simulink library "mylib"  (R2020a)
settings: Solver=VariableStepAuto  StartTime=0.0  StopTime=10.0  RelTol=1e-3
undefined symbols (not defined in the file): d_du_max_pu, dir_to_bus1, dir_to_bus_0L, dir_to_bus_2, dir_to_line1, dir_to_line_0L, dir_to_line_2, du_max_pu, du_ph_max_pu, Fi_0, Fi_T_H, Fi_T_L, Fi_T_M, I0_calc_0L, I0_comp_H, I0_comp_L, I0_comp_M, I0_max_0L, I2_max_2, I_diff1, I_diff2, I_diff3, I_diff4, I_diff5, I_diff_to, I_hight_CT1_G, I_hight_CT2_G, I_low_CT1, I_low_CT2, I_max1, I_max2, I_max3, I_max4, I_max5, I_min_sec_CT1, I_min_sec_CT2, I_unb, Iph_max_0L, Iph_max_2, jmp_in_zone, jmp_in_zone_0L, jmp_in_zone_2, K_dop, max_min1, only_K1_0L, only_K1_2, only_K2_0L, only_K2_2, only_K3_0L, only_K3_2, P_ctl_0, PQ_Fi_ctl_0, Q_ctl_0, S_set_0, set, set1, T_fast, T_I_ctl, T_off, T_on ... (+15)
libraries: $bdroot x184, powerlib_meascontrol x97
(part 6 of 14)

== system mylib/262_tnznp_line_st_v1/230_st18_ph/k_type ==
  In_a : Inport
  In_b : Inport  Port=2
  In_ c : Inport  Port=3
  only_K1 : Inport  Port=4
  only_K2 : Inport  Port=5
  only_K3 : Inport  Port=6
  1 : Switch  Criteria=u2 > Threshold
  Logical Operator{1,12,18..27} (12 alike) : Logic  Operator=NOT  AllPortsSameDT=off  OutDataTypeStr=boolean
  Logical Operator10 : Logic  AllPortsSameDT=off  OutDataTypeStr=boolean
  Logical Operator{2..4,7..8,11,14,17} (8 alike) : Logic  Inputs=3  AllPortsSameDT=off  OutDataTypeStr=boolean
  Logical Operator{5..6,13,16} (4 alike) : Logic  Operator=OR  Inputs=3  AllPortsSameDT=off  OutDataTypeStr=boolean
  Logical Operator15 : Logic  AllPortsSameDT=off  OutDataTypeStr=boolean
  Logical Operator9 : Logic  AllPortsSameDT=off  OutDataTypeStr=boolean
  out : Outport
  wires:
  In_ c/1 -> Logical Operator14/3, Logical Operator16/3, Logical Operator21/1, Logical Operator7/3, Logical Operator4/3, Logical Operator3/3, Logical Operator25/1, Logical Operator1/1
  Logical Operator16/1 -> 1/1
  Logical Operator13/1 -> 1/3
  1/1 -> out/1
  Logical Operator17/1 -> 1/2
  only_K3/1 -> Logical Operator20/1, Logical Operator15/1
  only_K2/1 -> Logical Operator10/1, Logical Operator18/1
  only_K1/1 -> Logical Operator9/1, Logical Operator19/1
  In_b/1 -> Logical Operator14/2, Logical Operator16/2, Logical Operator8/2, Logical Operator22/1, Logical Operator4/2, Logical Operator27/1, Logical Operator2/2, Logical Operator12/1
  Logical Operator27/1 -> Logical Operator3/2
  Logical Operator26/1 -> Logical Operator3/1
  Logical Operator25/1 -> Logical Operator2/3
  In_a/1 -> Logical Operator11/1, Logical Operator24/1, Logical Operator14/1, Logical Operator16/1, Logical Operator8/1, Logical Operator7/1, Logical Operator23/1, Logical Operator26/1
  Logical Operator24/1 -> Logical Operator2/1
  Logical Operator23/1 -> Logical Operator4/1
  Logical Operator22/1 -> Logical Operator7/2
  Logical Operator21/1 -> Logical Operator8/3
  Logical Operator20/1 -> Logical Operator17/3
  Logical Operator18/1 -> Logical Operator17/2
  Logical Operator19/1 -> Logical Operator17/1
  Logical Operator14/1 -> Logical Operator15/2
  Logical Operator15/1 -> Logical Operator13/3
  Logical Operator10/1 -> Logical Operator13/2
  Logical Operator9/1 -> Logical Operator13/1
  Logical Operator6/1 -> Logical Operator10/2
  Logical Operator5/1 -> Logical Operator9/2
  Logical Operator8/1 -> Logical Operator6/3
  Logical Operator7/1 -> Logical Operator6/2
  Logical Operator4/1 -> Logical Operator6/1
  Logical Operator3/1 -> Logical Operator5/3
  Logical Operator11/1 -> Logical Operator5/1
  Logical Operator2/1 -> Logical Operator5/2
  Logical Operator1/1 -> Logical Operator11/3
  Logical Operator12/1 -> Logical Operator11/2

== system mylib/264_DZ_trans_st_v1/Poly12_det19_ph/Za ==
  re : Inport
  im : Inport  Port=2
  Re1 : Inport  Port=3
  Im1 : Inport  Port=4
  Re2 : Inport  Port=5
  Im2 : Inport  Port=6
  Re3 : Inport  Port=7
  Im3 : Inport  Port=8
  Re4 : Inport  Port=9
  Im4 : Inport  Port=10
  Re5 : Inport  Port=11
  Im5 : Inport  Port=12
  Re6 : Inport  Port=13
  Im6 : Inport  Port=14
  Re7 : Inport  Port=15
  Im7 : Inport  Port=16
  Re8 : Inport  Port=17
  Im8 : Inport  Port=18
  Re9 : Inport  Port=19
  Im9 : Inport  Port=20
  Re10 : Inport  Port=21
  Im10 : Inport  Port=22
  Re11 : Inport  Port=23
  Im11 : Inport  Port=24
  Re12 : Inport  Port=25
  Im12 : Inport  Port=26
  Constant : Constant  Value=0
  Logical Operator : Logic  Operator=NOT  AllPortsSameDT=off  OutDataTypeStr=boolean
  Logical Operator1 : Logic  Operator=NOT  AllPortsSameDT=off  OutDataTypeStr=boolean
  stp_1 : Subsystem
  stp_10 : Subsystem
  stp_11 : Subsystem
  stp_12 : Subsystem
  stp_2 : Subsystem
  stp_3 : Subsystem
  stp_4 : Subsystem
  stp_5 : Subsystem
  stp_6 : Subsystem
  stp_7 : Subsystem
  stp_8 : Subsystem
  stp_9 : Subsystem
  Y : Outport
  not_Y : Outport  Port=2
  wires:
  Logical Operator/1 -> stp_1/9(start_pt)
  Constant/1 -> stp_1/1(Y_in), stp_1/2(alg_in), Logical Operator/1, stp_2/9(start_pt), stp_12/9(start_pt), stp_11/9(start_pt), stp_10/9(start_pt), stp_9/9(start_pt), stp_8/9(start_pt), stp_7/9(start_pt), stp_6/9(start_pt), stp_5/9(start_pt), stp_4/9(start_pt), stp_3/9(start_pt)
  stp_1/4(cur_Im) -> stp_2/4(Im_cur)
  stp_1/3(cur_Re) -> stp_2/3(Re_cur)
  stp_1/2(alg_out) -> stp_2/2(alg_in)
  stp_1/1(Y_out) -> stp_2/1(Y_in)
  im/1 -> stp_12/8(im), stp_11/8(im), stp_10/8(im), stp_9/8(im), stp_8/8(im), stp_7/8(im), stp_6/8(im), stp_5/8(im), stp_4/8(im), stp_3/8(im), stp_2/8(im), stp_1/8(im)
  re/1 -> stp_12/7(re), stp_11/7(re), stp_10/7(re), stp_9/7(re), stp_8/7(re), stp_7/7(re), stp_6/7(re), stp_5/7(re), stp_4/7(re), stp_3/7(re), stp_2/7(re), stp_1/7(re)
  Re1/1 -> stp_1/3(Re_cur), stp_1/10(Re_start), stp_12/5(Re_next), stp_12/10(Re_start), stp_11/10(Re_start), stp_10/10(Re_start), stp_9/10(Re_start), stp_8/10(Re_start), stp_7/10(Re_start), stp_6/10(Re_start), stp_5/10(Re_start), stp_4/10(Re_start), stp_3/10(Re_start), stp_2/10(Re_start)
  Im1/1 -> stp_1/4(Im_cur), stp_1/11(Im_start), stp_12/6(Im_next), stp_12/11(Im_start), stp_11/11(Im_start), stp_10/11(Im_start), stp_9/11(Im_start), stp_8/11(Im_start), stp_7/11(Im_start), stp_6/11(Im_start), stp_5/11(Im_start), stp_4/11(Im_start), stp_3/11(Im_start), stp_2/11(Im_start)
  Re2/1 -> stp_1/5(Re_next)
  Im2/1 -> stp_1/6(Im_next)
  Re3/1 -> stp_2/5(Re_next)
  Im3/1 -> stp_2/6(Im_next)
  Re4/1 -> stp_3/5(Re_next)
  Im4/1 -> stp_3/6(Im_next)
  stp_2/1(Y_out) -> stp_3/1(Y_in)
  stp_2/2(alg_out) -> stp_3/2(alg_in)
  stp_2/3(cur_Re) -> stp_3/3(Re_cur)
  stp_2/4(cur_Im) -> stp_3/4(Im_cur)
  stp_10/1(Y_out) -> stp_11/1(Y_in)
  stp_10/2(alg_out) -> stp_11/2(alg_in)
  stp_10/3(cur_Re) -> stp_11/3(Re_cur)
  stp_10/4(cur_Im) -> stp_11/4(Im_cur)
  stp_11/1(Y_out) -> stp_12/1(Y_in)
  stp_11/2(alg_out) -> stp_12/2(alg_in)
  stp_11/3(cur_Re) -> stp_12/3(Re_cur)
  stp_11/4(cur_Im) -> stp_12/4(Im_cur)
  stp_9/4(cur_Im) -> stp_10/4(Im_cur)
  stp_9/3(cur_Re) -> stp_10/3(Re_cur)
  stp_9/2(alg_out) -> stp_10/2(alg_in)
  stp_9/1(Y_out) -> stp_10/1(Y_in)
  stp_8/4(cur_Im) -> stp_9/4(Im_cur)
  stp_8/3(cur_Re) -> stp_9/3(Re_cur)
  stp_8/2(alg_out) -> stp_9/2(alg_in)
  stp_8/1(Y_out) -> stp_9/1(Y_in)
  stp_7/4(cur_Im) -> stp_8/4(Im_cur)
  stp_7/3(cur_Re) -> stp_8/3(Re_cur)
  stp_7/2(alg_out) -> stp_8/2(alg_in)
  stp_7/1(Y_out) -> stp_8/1(Y_in)
  stp_6/4(cur_Im) -> stp_7/4(Im_cur)
  stp_6/3(cur_Re) -> stp_7/3(Re_cur)
  stp_6/2(alg_out) -> stp_7/2(alg_in)
  stp_6/1(Y_out) -> stp_7/1(Y_in)
  stp_5/4(cur_Im) -> stp_6/4(Im_cur)
  stp_5/3(cur_Re) -> stp_6/3(Re_cur)
  stp_5/2(alg_out) -> stp_6/2(alg_in)
  stp_5/1(Y_out) -> stp_6/1(Y_in)
  stp_4/4(cur_Im) -> stp_5/4(Im_cur)
  stp_4/3(cur_Re) -> stp_5/3(Re_cur)
  stp_4/2(alg_out) -> stp_5/2(alg_in)
  stp_4/1(Y_out) -> stp_5/1(Y_in)
  stp_3/4(cur_Im) -> stp_4/4(Im_cur)
  stp_3/3(cur_Re) -> stp_4/3(Re_cur)
  stp_3/2(alg_out) -> stp_4/2(alg_in)
  stp_3/1(Y_out) -> stp_4/1(Y_in)
  Re5/1 -> stp_4/5(Re_next)
  Im5/1 -> stp_4/6(Im_next)
  Re6/1 -> stp_5/5(Re_next)
  Im6/1 -> stp_5/6(Im_next)
  Re7/1 -> stp_6/5(Re_next)
  Im7/1 -> stp_6/6(Im_next)
  Re8/1 -> stp_7/5(Re_next)
  Im8/1 -> stp_7/6(Im_next)
  Re9/1 -> stp_8/5(Re_next)
  Im9/1 -> stp_8/6(Im_next)
  Re10/1 -> stp_9/5(Re_next)
  Im10/1 -> stp_9/6(Im_next)
  Re11/1 -> stp_10/5(Re_next)
  Im11/1 -> stp_10/6(Im_next)
  Re12/1 -> stp_11/5(Re_next)
  Im12/1 -> stp_11/6(Im_next)
  stp_12/1(Y_out) -> Logical Operator1/1, Y/1
  Logical Operator1/1 -> not_Y/1

== system mylib/264_DZ_trans_st_v1/Poly12_det19_ph/Zb ==
  re : Inport
  im : Inport  Port=2
  Re1 : Inport  Port=3
  Im1 : Inport  Port=4
  Re2 : Inport  Port=5
  Im2 : Inport  Port=6
  Re3 : Inport  Port=7
  Im3 : Inport  Port=8
  Re4 : Inport  Port=9
  Im4 : Inport  Port=10
  Re5 : Inport  Port=11
  Im5 : Inport  Port=12
  Re6 : Inport  Port=13
  Im6 : Inport  Port=14
  Re7 : Inport  Port=15
  Im7 : Inport  Port=16
  Re8 : Inport  Port=17
  Im8 : Inport  Port=18
  Re9 : Inport  Port=19
  Im9 : Inport  Port=20
  Re10 : Inport  Port=21
  Im10 : Inport  Port=22
  Re11 : Inport  Port=23
  Im11 : Inport  Port=24
  Re12 : Inport  Port=25
  Im12 : Inport  Port=26
  Constant : Constant  Value=0
  Logical Operator : Logic  Operator=NOT  AllPortsSameDT=off  OutDataTypeStr=boolean
  Logical Operator1 : Logic  Operator=NOT  AllPortsSameDT=off  OutDataTypeStr=boolean
  stp_1 : Subsystem
  stp_10 : Subsystem
  stp_11 : Subsystem
  stp_12 : Subsystem
  stp_2 : Subsystem
  stp_3 : Subsystem
  stp_4 : Subsystem
  stp_5 : Subsystem
  stp_6 : Subsystem
  stp_7 : Subsystem
  stp_8 : Subsystem
  stp_9 : Subsystem
  Y : Outport
  not_Y : Outport  Port=2
  wires:
  Logical Operator/1 -> stp_1/9(start_pt)
  Constant/1 -> stp_1/1(Y_in), stp_1/2(alg_in), Logical Operator/1, stp_2/9(start_pt), stp_12/9(start_pt), stp_11/9(start_pt), stp_10/9(start_pt), stp_9/9(start_pt), stp_8/9(start_pt), stp_7/9(start_pt), stp_6/9(start_pt), stp_5/9(start_pt), stp_4/9(start_pt), stp_3/9(start_pt)
  stp_1/4(cur_Im) -> stp_2/4(Im_cur)
  stp_1/3(cur_Re) -> stp_2/3(Re_cur)
  stp_1/2(alg_out) -> stp_2/2(alg_in)
  stp_1/1(Y_out) -> stp_2/1(Y_in)
  im/1 -> stp_12/8(im), stp_11/8(im), stp_10/8(im), stp_9/8(im), stp_8/8(im), stp_7/8(im), stp_6/8(im), stp_5/8(im), stp_4/8(im), stp_3/8(im), stp_2/8(im), stp_1/8(im)
  re/1 -> stp_12/7(re), stp_11/7(re), stp_10/7(re), stp_9/7(re), stp_8/7(re), stp_7/7(re), stp_6/7(re), stp_5/7(re), stp_4/7(re), stp_3/7(re), stp_2/7(re), stp_1/7(re)
  Re1/1 -> stp_1/3(Re_cur), stp_1/10(Re_start), stp_12/5(Re_next), stp_12/10(Re_start), stp_11/10(Re_start), stp_10/10(Re_start), stp_9/10(Re_start), stp_8/10(Re_start), stp_7/10(Re_start), stp_6/10(Re_start), stp_5/10(Re_start), stp_4/10(Re_start), stp_3/10(Re_start), stp_2/10(Re_start)
  Im1/1 -> stp_1/4(Im_cur), stp_1/11(Im_start), stp_12/6(Im_next), stp_12/11(Im_start), stp_11/11(Im_start), stp_10/11(Im_start), stp_9/11(Im_start), stp_8/11(Im_start), stp_7/11(Im_start), stp_6/11(Im_start), stp_5/11(Im_start), stp_4/11(Im_start), stp_3/11(Im_start), stp_2/11(Im_start)
  Re2/1 -> stp_1/5(Re_next)
  Im2/1 -> stp_1/6(Im_next)
  Re3/1 -> stp_2/5(Re_next)
  Im3/1 -> stp_2/6(Im_next)
  Re4/1 -> stp_3/5(Re_next)
  Im4/1 -> stp_3/6(Im_next)
  stp_2/1(Y_out) -> stp_3/1(Y_in)
  stp_2/2(alg_out) -> stp_3/2(alg_in)
  stp_2/3(cur_Re) -> stp_3/3(Re_cur)
  stp_2/4(cur_Im) -> stp_3/4(Im_cur)
  stp_10/1(Y_out) -> stp_11/1(Y_in)
  stp_10/2(alg_out) -> stp_11/2(alg_in)
  stp_10/3(cur_Re) -> stp_11/3(Re_cur)
  stp_10/4(cur_Im) -> stp_11/4(Im_cur)
  stp_11/1(Y_out) -> stp_12/1(Y_in)
  stp_11/2(alg_out) -> stp_12/2(alg_in)
  stp_11/3(cur_Re) -> stp_12/3(Re_cur)
  stp_11/4(cur_Im) -> stp_12/4(Im_cur)
  stp_9/4(cur_Im) -> stp_10/4(Im_cur)
  stp_9/3(cur_Re) -> stp_10/3(Re_cur)
  stp_9/2(alg_out) -> stp_10/2(alg_in)
  stp_9/1(Y_out) -> stp_10/1(Y_in)
  stp_8/4(cur_Im) -> stp_9/4(Im_cur)
  stp_8/3(cur_Re) -> stp_9/3(Re_cur)
  stp_8/2(alg_out) -> stp_9/2(alg_in)
  stp_8/1(Y_out) -> stp_9/1(Y_in)
  stp_7/4(cur_Im) -> stp_8/4(Im_cur)
  stp_7/3(cur_Re) -> stp_8/3(Re_cur)
  stp_7/2(alg_out) -> stp_8/2(alg_in)
  stp_7/1(Y_out) -> stp_8/1(Y_in)
  stp_6/4(cur_Im) -> stp_7/4(Im_cur)
  stp_6/3(cur_Re) -> stp_7/3(Re_cur)
  stp_6/2(alg_out) -> stp_7/2(alg_in)
  stp_6/1(Y_out) -> stp_7/1(Y_in)
  stp_5/4(cur_Im) -> stp_6/4(Im_cur)
  stp_5/3(cur_Re) -> stp_6/3(Re_cur)
  stp_5/2(alg_out) -> stp_6/2(alg_in)
  stp_5/1(Y_out) -> stp_6/1(Y_in)
  stp_4/4(cur_Im) -> stp_5/4(Im_cur)
  stp_4/3(cur_Re) -> stp_5/3(Re_cur)
  stp_4/2(alg_out) -> stp_5/2(alg_in)
  stp_4/1(Y_out) -> stp_5/1(Y_in)
  stp_3/4(cur_Im) -> stp_4/4(Im_cur)
  stp_3/3(cur_Re) -> stp_4/3(Re_cur)
  stp_3/2(alg_out) -> stp_4/2(alg_in)
  stp_3/1(Y_out) -> stp_4/1(Y_in)
  Re5/1 -> stp_4/5(Re_next)
  Im5/1 -> stp_4/6(Im_next)
  Re6/1 -> stp_5/5(Re_next)
  Im6/1 -> stp_5/6(Im_next)
  Re7/1 -> stp_6/5(Re_next)
  Im7/1 -> stp_6/6(Im_next)
  Re8/1 -> stp_7/5(Re_next)
  Im8/1 -> stp_7/6(Im_next)
  Re9/1 -> stp_8/5(Re_next)
  Im9/1 -> stp_8/6(Im_next)
  Re10/1 -> stp_9/5(Re_next)
  Im10/1 -> stp_9/6(Im_next)
  Re11/1 -> stp_10/5(Re_next)
  Im11/1 -> stp_10/6(Im_next)
  Re12/1 -> stp_11/5(Re_next)
  Im12/1 -> stp_11/6(Im_next)
  stp_12/1(Y_out) -> Logical Operator1/1, Y/1
  Logical Operator1/1 -> not_Y/1

== system mylib/264_DZ_trans_st_v1/Poly12_det19_ph/Zc ==
  re : Inport
  im : Inport  Port=2
  Re1 : Inport  Port=3
  Im1 : Inport  Port=4
  Re2 : Inport  Port=5
  Im2 : Inport  Port=6
  Re3 : Inport  Port=7
  Im3 : Inport  Port=8
  Re4 : Inport  Port=9
  Im4 : Inport  Port=10
  Re5 : Inport  Port=11
  Im5 : Inport  Port=12
  Re6 : Inport  Port=13
  Im6 : Inport  Port=14
  Re7 : Inport  Port=15
  Im7 : Inport  Port=16
  Re8 : Inport  Port=17
  Im8 : Inport  Port=18
  Re9 : Inport  Port=19
  Im9 : Inport  Port=20
  Re10 : Inport  Port=21
  Im10 : Inport  Port=22
  Re11 : Inport  Port=23
  Im11 : Inport  Port=24
  Re12 : Inport  Port=25
  Im12 : Inport  Port=26
  Constant : Constant  Value=0
  Logical Operator : Logic  Operator=NOT  AllPortsSameDT=off  OutDataTypeStr=boolean
  Logical Operator1 : Logic  Operator=NOT  AllPortsSameDT=off  OutDataTypeStr=boolean
  stp_1 : Subsystem
  stp_10 : Subsystem
  stp_11 : Subsystem
  stp_12 : Subsystem
  stp_2 : Subsystem
  stp_3 : Subsystem
  stp_4 : Subsystem
  stp_5 : Subsystem
  stp_6 : Subsystem
  stp_7 : Subsystem
  stp_8 : Subsystem
  stp_9 : Subsystem
  Y : Outport
  not_Y : Outport  Port=2
  wires:
  Logical Operator/1 -> stp_1/9(start_pt)
  Constant/1 -> stp_1/1(Y_in), stp_1/2(alg_in), Logical Operator/1, stp_2/9(start_pt), stp_12/9(start_pt), stp_11/9(start_pt), stp_10/9(start_pt), stp_9/9(start_pt), stp_8/9(start_pt), stp_7/9(start_pt), stp_6/9(start_pt), stp_5/9(start_pt), stp_4/9(start_pt), stp_3/9(start_pt)
  stp_1/4(cur_Im) -> stp_2/4(Im_cur)
  stp_1/3(cur_Re) -> stp_2/3(Re_cur)
  stp_1/2(alg_out) -> stp_2/2(alg_in)
  stp_1/1(Y_out) -> stp_2/1(Y_in)
  im/1 -> stp_12/8(im), stp_11/8(im), stp_10/8(im), stp_9/8(im), stp_8/8(im), stp_7/8(im), stp_6/8(im), stp_5/8(im), stp_4/8(im), stp_3/8(im), stp_2/8(im), stp_1/8(im)
  re/1 -> stp_12/7(re), stp_11/7(re), stp_10/7(re), stp_9/7(re), stp_8/7(re), stp_7/7(re), stp_6/7(re), stp_5/7(re), stp_4/7(re), stp_3/7(re), stp_2/7(re), stp_1/7(re)
  Re1/1 -> stp_1/3(Re_cur), stp_1/10(Re_start), stp_12/5(Re_next), stp_12/10(Re_start), stp_11/10(Re_start), stp_10/10(Re_start), stp_9/10(Re_start), stp_8/10(Re_start), stp_7/10(Re_start), stp_6/10(Re_start), stp_5/10(Re_start), stp_4/10(Re_start), stp_3/10(Re_start), stp_2/10(Re_start)
  Im1/1 -> stp_1/4(Im_cur), stp_1/11(Im_start), stp_12/6(Im_next), stp_12/11(Im_start), stp_11/11(Im_start), stp_10/11(Im_start), stp_9/11(Im_start), stp_8/11(Im_start), stp_7/11(Im_start), stp_6/11(Im_start), stp_5/11(Im_start), stp_4/11(Im_start), stp_3/11(Im_start), stp_2/11(Im_start)
  Re2/1 -> stp_1/5(Re_next)
  Im2/1 -> stp_1/6(Im_next)
  Re3/1 -> stp_2/5(Re_next)
  Im3/1 -> stp_2/6(Im_next)
  Re4/1 -> stp_3/5(Re_next)
  Im4/1 -> stp_3/6(Im_next)
  stp_2/1(Y_out) -> stp_3/1(Y_in)
  stp_2/2(alg_out) -> stp_3/2(alg_in)
  stp_2/3(cur_Re) -> stp_3/3(Re_cur)
  stp_2/4(cur_Im) -> stp_3/4(Im_cur)
  stp_10/1(Y_out) -> stp_11/1(Y_in)
  stp_10/2(alg_out) -> stp_11/2(alg_in)
  stp_10/3(cur_Re) -> stp_11/3(Re_cur)
  stp_10/4(cur_Im) -> stp_11/4(Im_cur)
  stp_11/1(Y_out) -> stp_12/1(Y_in)
  stp_11/2(alg_out) -> stp_12/2(alg_in)
  stp_11/3(cur_Re) -> stp_12/3(Re_cur)
  stp_11/4(cur_Im) -> stp_12/4(Im_cur)
  stp_9/4(cur_Im) -> stp_10/4(Im_cur)
  stp_9/3(cur_Re) -> stp_10/3(Re_cur)
  stp_9/2(alg_out) -> stp_10/2(alg_in)
  stp_9/1(Y_out) -> stp_10/1(Y_in)
  stp_8/4(cur_Im) -> stp_9/4(Im_cur)
  stp_8/3(cur_Re) -> stp_9/3(Re_cur)
  stp_8/2(alg_out) -> stp_9/2(alg_in)
  stp_8/1(Y_out) -> stp_9/1(Y_in)
  stp_7/4(cur_Im) -> stp_8/4(Im_cur)
  stp_7/3(cur_Re) -> stp_8/3(Re_cur)
  stp_7/2(alg_out) -> stp_8/2(alg_in)
  stp_7/1(Y_out) -> stp_8/1(Y_in)
  stp_6/4(cur_Im) -> stp_7/4(Im_cur)
  stp_6/3(cur_Re) -> stp_7/3(Re_cur)
  stp_6/2(alg_out) -> stp_7/2(alg_in)
  stp_6/1(Y_out) -> stp_7/1(Y_in)
  stp_5/4(cur_Im) -> stp_6/4(Im_cur)
  stp_5/3(cur_Re) -> stp_6/3(Re_cur)
  stp_5/2(alg_out) -> stp_6/2(alg_in)
  stp_5/1(Y_out) -> stp_6/1(Y_in)
  stp_4/4(cur_Im) -> stp_5/4(Im_cur)
  stp_4/3(cur_Re) -> stp_5/3(Re_cur)
  stp_4/2(alg_out) -> stp_5/2(alg_in)
  stp_4/1(Y_out) -> stp_5/1(Y_in)
  stp_3/4(cur_Im) -> stp_4/4(Im_cur)
  stp_3/3(cur_Re) -> stp_4/3(Re_cur)
  stp_3/2(alg_out) -> stp_4/2(alg_in)
  stp_3/1(Y_out) -> stp_4/1(Y_in)
  Re5/1 -> stp_4/5(Re_next)
  Im5/1 -> stp_4/6(Im_next)
  Re6/1 -> stp_5/5(Re_next)
  Im6/1 -> stp_5/6(Im_next)
  Re7/1 -> stp_6/5(Re_next)
  Im7/1 -> stp_6/6(Im_next)
  Re8/1 -> stp_7/5(Re_next)
  Im8/1 -> stp_7/6(Im_next)
  Re9/1 -> stp_8/5(Re_next)
  Im9/1 -> stp_8/6(Im_next)
  Re10/1 -> stp_9/5(Re_next)
  Im10/1 -> stp_9/6(Im_next)
  Re11/1 -> stp_10/5(Re_next)
  Im11/1 -> stp_10/6(Im_next)
  Re12/1 -> stp_11/5(Re_next)
  Im12/1 -> stp_11/6(Im_next)
  stp_12/1(Y_out) -> Logical Operator1/1, Y/1
  Logical Operator1/1 -> not_Y/1

== system mylib/264_DZ_trans_st_v1/St1/Subsystem ==
  T_fast_time : Inport
  T_fast_zero : Inport  Port=2
  "In1 " : Inport  Port=3
  "In2 " : Inport  Port=4
  "In3 " : Inport  Port=5
  {1..5,7} (6 alike) : Switch  Criteria=u2 > Threshold
  T1 : powerlib_meascontrol/Logic/On Delay  DelayType=On delay  delay=T_st  ic=0  Ts=0
  T2 : powerlib_meascontrol/Logic/On Delay  DelayType=On delay  delay=T_st  ic=0  Ts=0
  T3 : powerlib_meascontrol/Logic/On Delay  DelayType=On delay  delay=T_st  ic=0  Ts=0
  T4 : powerlib_meascontrol/Logic/On Delay  DelayType=On delay  delay=T_fast  ic=0  Ts=0
  T5 : powerlib_meascontrol/Logic/On Delay  DelayType=On delay  delay=T_fast  ic=0  Ts=0
  T6 : powerlib_meascontrol/Logic/On Delay  DelayType=On delay  delay=T_fast  ic=0  Ts=0
  T7 : powerlib_meascontrol/Logic/On Delay  DelayType=Off delay  delay=T_fast  ic=0  Ts=0
  Out1 : Outport
  Out2 : Outport  Port=2
  Out3 : Outport  Port=3
  wires:
  "In3 "/1 -> T4/1, T2/1, 4/1
  "In2 "/1 -> 3/1, T5/1, T1/1
  "In1 "/1 -> 5/1, T3/1, T6/1
  T7/1 -> 2/2, 1/2, 7/2
  T_fast_time/1 -> T7/1
  T4/1 -> 2/1
  T5/1 -> 1/1
  T6/1 -> 7/1
  T3/1 -> 7/3
  T1/1 -> 1/3
  T2/1 -> 2/3
  T_fast_zero/1 -> 5/2, 3/2, 4/2
  7/1 -> 5/3
  1/1 -> 3/3
  2/1 -> 4/3
  5/1 -> Out1/1
  3/1 -> Out2/1
  4/1 -> Out3/1

== system mylib/264_DZ_trans_st_v1/St1/in_1 ==
  jmp_in_zone : Inport
  in : Inport  Port=2
  jmp : Inport  Port=3
  1 : Switch  Criteria=u2 > Threshold
  10 : Logic  AllPortsSameDT=off  OutDataTypeStr=boolean
  11 : Logic  Operator=NOT  AllPortsSameDT=off  OutDataTypeStr=boolean
  12 : Memory
  3 : Logic  AllPortsSameDT=off  OutDataTypeStr=boolean
  RS : $bdroot/RS  SystemSampleTime=-1  Latency=0  AutoFrameSizeCalculation=off
  R_TRIG : $bdroot/R_TRIG  SystemSampleTime=-1  Latency=0  AutoFrameSizeCalculation=off
  T1 : powerlib_meascontrol/Logic/On Delay  DelayType=Off delay  delay=T_reset  ic=0  Ts=0
  T2 : powerlib_meascontrol/Logic/On Delay  DelayType=On delay  delay=T_reset  ic=0  Ts=0
  Y : Outport
  wires:
  RS/1 -> 12/1, Y/1
  in/1 -> 11/1, R_TRIG/1, 1/3
  R_TRIG/1 -> 1/1
  jmp_in_zone/1 -> 1/2
  11/1 -> 10/2
  10/1 -> T2/1
  T1/1 -> 3/2
  1/1 -> 3/1
  jmp/1 -> T1/1
  12/1 -> 10/1
  T2/1 -> RS/2
  3/1 -> RS/1

== system mylib/264_DZ_trans_st_v1/St1/in_2 ==
  jmp_in_zone : Inport
  in : Inport  Port=2
  jmp : Inport  Port=3
  1 : Switch  Criteria=u2 > Threshold
  10 : Logic  AllPortsSameDT=off  OutDataTypeStr=boolean
  11 : Logic  Operator=NOT  AllPortsSameDT=off  OutDataTypeStr=boolean
  12 : Memory
  3 : Logic  AllPortsSameDT=off  OutDataTypeStr=boolean
  RS : $bdroot/RS  SystemSampleTime=-1  Latency=0  AutoFrameSizeCalculation=off
  R_TRIG : $bdroot/R_TRIG  SystemSampleTime=-1  Latency=0  AutoFrameSizeCalculation=off
  T1 : powerlib_meascontrol/Logic/On Delay  DelayType=Off delay  delay=T_reset  ic=0  Ts=0
  T2 : powerlib_meascontrol/Logic/On Delay  DelayType=On delay  delay=T_reset  ic=0  Ts=0
  Y : Outport
  wires:
  RS/1 -> 12/1, Y/1
  in/1 -> 11/1, R_TRIG/1, 1/3
  R_TRIG/1 -> 1/1
  jmp_in_zone/1 -> 1/2
  11/1 -> 10/2
  10/1 -> T2/1
  T1/1 -> 3/2
  1/1 -> 3/1
  jmp/1 -> T1/1
  12/1 -> 10/1
  T2/1 -> RS/2
  3/1 -> RS/1

== system mylib/264_DZ_trans_st_v1/St1/in_3 ==
  jmp_in_zone : Inport
  in : Inport  Port=2
  jmp : Inport  Port=3
  1 : Switch  Criteria=u2 > Threshold
  10 : Logic  AllPortsSameDT=off  OutDataTypeStr=boolean
  11 : Logic  Operator=NOT  AllPortsSameDT=off  OutDataTypeStr=boolean
  12 : Memory
  3 : Logic  AllPortsSameDT=off  OutDataTypeStr=boolean
  RS : $bdroot/RS  SystemSampleTime=-1  Latency=0  AutoFrameSizeCalculation=off
  R_TRIG : $bdroot/R_TRIG  SystemSampleTime=-1  Latency=0  AutoFrameSizeCalculation=off
  T1 : powerlib_meascontrol/Logic/On Delay  DelayType=Off delay  delay=T_reset  ic=0  Ts=0
  T2 : powerlib_meascontrol/Logic/On Delay  DelayType=On delay  delay=T_reset  ic=0  Ts=0
  Y : Outport
  wires:
  RS/1 -> 12/1, Y/1
  in/1 -> 11/1, R_TRIG/1, 1/3
  R_TRIG/1 -> 1/1
  jmp_in_zone/1 -> 1/2
  11/1 -> 10/2
  10/1 -> T2/1
  T1/1 -> 3/2
  1/1 -> 3/1
  jmp/1 -> T1/1
  12/1 -> 10/1
  T2/1 -> RS/2
  3/1 -> RS/1

== system mylib/264_DZ_trans_st_v1/St1/k_type ==
  In_a : Inport
  In_b : Inport  Port=2
  In_ c : Inport  Port=3
  only_K1 : Inport  Port=4
  only_K2 : Inport  Port=5
  only_K3 : Inport  Port=6
  1 : Switch  Criteria=u2 > Threshold
  Logical Operator{1,12,18..27} (12 alike) : Logic  Operator=NOT  AllPortsSameDT=off  OutDataTypeStr=boolean
  Logical Operator10 : Logic  AllPortsSameDT=off  OutDataTypeStr=boolean
  Logical Operator{2..4,7..8,11,14,17} (8 alike) : Logic  Inputs=3  AllPortsSameDT=off  OutDataTypeStr=boolean
  Logical Operator{5..6,13,16} (4 alike) : Logic  Operator=OR  Inputs=3  AllPortsSameDT=off  OutDataTypeStr=boolean
  Logical Operator15 : Logic  AllPortsSameDT=off  OutDataTypeStr=boolean
  Logical Operator9 : Logic  AllPortsSameDT=off  OutDataTypeStr=boolean
  out : Outport
  wires:
  Logical Operator12/1 -> Logical Operator11/2
  Logical Operator1/1 -> Logical Operator11/3
  Logical Operator2/1 -> Logical Operator5/2
  Logical Operator11/1 -> Logical Operator5/1
  Logical Operator3/1 -> Logical Operator5/3
  Logical Operator4/1 -> Logical Operator6/1
  Logical Operator7/1 -> Logical Operator6/2
  Logical Operator8/1 -> Logical Operator6/3
  Logical Operator5/1 -> Logical Operator9/2
  Logical Operator6/1 -> Logical Operator10/2
  Logical Operator9/1 -> Logical Operator13/1
  Logical Operator10/1 -> Logical Operator13/2
  Logical Operator15/1 -> Logical Operator13/3
  Logical Operator14/1 -> Logical Operator15/2
  Logical Operator19/1 -> Logical Operator17/1
  Logical Operator18/1 -> Logical Operator17/2
  Logical Operator20/1 -> Logical Operator17/3
  Logical Operator21/1 -> Logical Operator8/3
  Logical Operator22/1 -> Logical Operator7/2
  Logical Operator23/1 -> Logical Operator4/1
  Logical Operator24/1 -> Logical Operator2/1
  In_a/1 -> Logical Operator26/1, Logical Operator23/1, Logical Operator7/1, Logical Operator8/1, Logical Operator16/1, Logical Operator14/1, Logical Operator24/1, Logical Operator11/1
  Logical Operator25/1 -> Logical Operator2/3
  Logical Operator26/1 -> Logical Operator3/1
  Logical Operator27/1 -> Logical Operator3/2
  In_b/1 -> Logical Operator12/1, Logical Operator2/2, Logical Operator27/1, Logical Operator4/2, Logical Operator22/1, Logical Operator8/2, Logical Operator16/2, Logical Operator14/2
  only_K1/1 -> Logical Operator19/1, Logical Operator9/1
  only_K2/1 -> Logical Operator18/1, Logical Operator10/1
  only_K3/1 -> Logical Operator15/1, Logical Operator20/1
  Logical Operator17/1 -> 1/2
  1/1 -> out/1
  Logical Operator13/1 -> 1/3
  Logical Operator16/1 -> 1/1
  In_ c/1 -> Logical Operator1/1, Logical Operator25/1, Logical Operator3/3, Logical Operator4/3, Logical Operator7/3, Logical Operator21/1, Logical Operator16/3, Logical Operator14/3

== system mylib/264_DZ_trans_st_v1/St2/Subsystem ==
  T_fast_time : Inport
  T_fast_zero : Inport  Port=2
  "In1 " : Inport  Port=3
  "In2 " : Inport  Port=4
  "In3 " : Inport  Port=5
  {1..5,7} (6 alike) : Switch  Criteria=u2 > Threshold
  T1 : powerlib_meascontrol/Logic/On Delay  DelayType=On delay  delay=T_st  ic=0  Ts=0
  T2 : powerlib_meascontrol/Logic/On Delay  DelayType=On delay  delay=T_st  ic=0  Ts=0
  T3 : powerlib_meascontrol/Logic/On Delay  DelayType=On delay  delay=T_st  ic=0  Ts=0
  T4 : powerlib_meascontrol/Logic/On Delay  DelayType=On delay  delay=T_fast  ic=0  Ts=0
  T5 : powerlib_meascontrol/Logic/On Delay  DelayType=On delay  delay=T_fast  ic=0  Ts=0
  T6 : powerlib_meascontrol/Logic/On Delay  DelayType=On delay  delay=T_fast  ic=0  Ts=0
  T7 : powerlib_meascontrol/Logic/On Delay  DelayType=Off delay  delay=T_fast  ic=0  Ts=0
  Out1 : Outport
  Out2 : Outport  Port=2
  Out3 : Outport  Port=3
  wires:
  "In3 "/1 -> T4/1, T2/1, 4/1
  "In2 "/1 -> 3/1, T5/1, T1/1
  "In1 "/1 -> 5/1, T3/1, T6/1
  T7/1 -> 2/2, 1/2, 7/2
  T_fast_time/1 -> T7/1
  T4/1 -> 2/1
  T5/1 -> 1/1
  T6/1 -> 7/1
  T3/1 -> 7/3
  T1/1 -> 1/3
  T2/1 -> 2/3
  T_fast_zero/1 -> 5/2, 3/2, 4/2
  7/1 -> 5/3
  1/1 -> 3/3
  2/1 -> 4/3
  5/1 -> Out1/1
  3/1 -> Out2/1
  4/1 -> Out3/1

== system mylib/264_DZ_trans_st_v1/St2/in_1 ==
  jmp_in_zone : Inport
  in : Inport  Port=2
  jmp : Inport  Port=3
  1 : Switch  Criteria=u2 > Threshold
  10 : Logic  AllPortsSameDT=off  OutDataTypeStr=boolean
  11 : Logic  Operator=NOT  AllPortsSameDT=off  OutDataTypeStr=boolean
  12 : Memory
  3 : Logic  AllPortsSameDT=off  OutDataTypeStr=boolean
  RS : $bdroot/RS  SystemSampleTime=-1  Latency=0  AutoFrameSizeCalculation=off
  R_TRIG : $bdroot/R_TRIG  SystemSampleTime=-1  Latency=0  AutoFrameSizeCalculation=off
  T1 : powerlib_meascontrol/Logic/On Delay  DelayType=Off delay  delay=T_reset  ic=0  Ts=0
  T2 : powerlib_meascontrol/Logic/On Delay  DelayType=On delay  delay=T_reset  ic=0  Ts=0
  Y : Outport
  wires:
  RS/1 -> 12/1, Y/1
  in/1 -> 11/1, R_TRIG/1, 1/3
  R_TRIG/1 -> 1/1
  jmp_in_zone/1 -> 1/2
  11/1 -> 10/2
  10/1 -> T2/1
  T1/1 -> 3/2
  1/1 -> 3/1
  jmp/1 -> T1/1
  12/1 -> 10/1
  T2/1 -> RS/2
  3/1 -> RS/1

== system mylib/264_DZ_trans_st_v1/St2/in_2 ==
  jmp_in_zone : Inport
  in : Inport  Port=2
  jmp : Inport  Port=3
  1 : Switch  Criteria=u2 > Threshold
  10 : Logic  AllPortsSameDT=off  OutDataTypeStr=boolean
  11 : Logic  Operator=NOT  AllPortsSameDT=off  OutDataTypeStr=boolean
  12 : Memory
  3 : Logic  AllPortsSameDT=off  OutDataTypeStr=boolean
  RS : $bdroot/RS  SystemSampleTime=-1  Latency=0  AutoFrameSizeCalculation=off
  R_TRIG : $bdroot/R_TRIG  SystemSampleTime=-1  Latency=0  AutoFrameSizeCalculation=off
  T1 : powerlib_meascontrol/Logic/On Delay  DelayType=Off delay  delay=T_reset  ic=0  Ts=0
  T2 : powerlib_meascontrol/Logic/On Delay  DelayType=On delay  delay=T_reset  ic=0  Ts=0
  Y : Outport
  wires:
  RS/1 -> 12/1, Y/1
  in/1 -> 11/1, R_TRIG/1, 1/3
  R_TRIG/1 -> 1/1
  jmp_in_zone/1 -> 1/2
  11/1 -> 10/2
  10/1 -> T2/1
  T1/1 -> 3/2
  1/1 -> 3/1
  jmp/1 -> T1/1
  12/1 -> 10/1
  T2/1 -> RS/2
  3/1 -> RS/1

== system mylib/264_DZ_trans_st_v1/St2/in_3 ==
  jmp_in_zone : Inport
  in : Inport  Port=2
  jmp : Inport  Port=3
  1 : Switch  Criteria=u2 > Threshold
  10 : Logic  AllPortsSameDT=off  OutDataTypeStr=boolean
  11 : Logic  Operator=NOT  AllPortsSameDT=off  OutDataTypeStr=boolean
  12 : Memory
  3 : Logic  AllPortsSameDT=off  OutDataTypeStr=boolean
  RS : $bdroot/RS  SystemSampleTime=-1  Latency=0  AutoFrameSizeCalculation=off
  R_TRIG : $bdroot/R_TRIG  SystemSampleTime=-1  Latency=0  AutoFrameSizeCalculation=off
  T1 : powerlib_meascontrol/Logic/On Delay  DelayType=Off delay  delay=T_reset  ic=0  Ts=0
  T2 : powerlib_meascontrol/Logic/On Delay  DelayType=On delay  delay=T_reset  ic=0  Ts=0
  Y : Outport
  wires:
  RS/1 -> 12/1, Y/1
  in/1 -> 11/1, R_TRIG/1, 1/3
  R_TRIG/1 -> 1/1
  jmp_in_zone/1 -> 1/2
  11/1 -> 10/2
  10/1 -> T2/1
  T1/1 -> 3/2
  1/1 -> 3/1
  jmp/1 -> T1/1
  12/1 -> 10/1
  T2/1 -> RS/2
  3/1 -> RS/1

== system mylib/264_DZ_trans_st_v1/St2/k_type ==
  In_a : Inport
  In_b : Inport  Port=2
  In_ c : Inport  Port=3
  only_K1 : Inport  Port=4
  only_K2 : Inport  Port=5
  only_K3 : Inport  Port=6
  1 : Switch  Criteria=u2 > Threshold
  Logical Operator{1,12,18..27} (12 alike) : Logic  Operator=NOT  AllPortsSameDT=off  OutDataTypeStr=boolean
  Logical Operator10 : Logic  AllPortsSameDT=off  OutDataTypeStr=boolean
  Logical Operator{2..4,7..8,11,14,17} (8 alike) : Logic  Inputs=3  AllPortsSameDT=off  OutDataTypeStr=boolean
  Logical Operator{5..6,13,16} (4 alike) : Logic  Operator=OR  Inputs=3  AllPortsSameDT=off  OutDataTypeStr=boolean
  Logical Operator15 : Logic  AllPortsSameDT=off  OutDataTypeStr=boolean
  Logical Operator9 : Logic  AllPortsSameDT=off  OutDataTypeStr=boolean
  out : Outport
  wires:
  Logical Operator12/1 -> Logical Operator11/2
  Logical Operator1/1 -> Logical Operator11/3
  Logical Operator2/1 -> Logical Operator5/2
  Logical Operator11/1 -> Logical Operator5/1
  Logical Operator3/1 -> Logical Operator5/3
  Logical Operator4/1 -> Logical Operator6/1
  Logical Operator7/1 -> Logical Operator6/2
  Logical Operator8/1 -> Logical Operator6/3
  Logical Operator5/1 -> Logical Operator9/2
  Logical Operator6/1 -> Logical Operator10/2
  Logical Operator9/1 -> Logical Operator13/1
  Logical Operator10/1 -> Logical Operator13/2
  Logical Operator15/1 -> Logical Operator13/3
  Logical Operator14/1 -> Logical Operator15/2
  Logical Operator19/1 -> Logical Operator17/1
  Logical Operator18/1 -> Logical Operator17/2
  Logical Operator20/1 -> Logical Operator17/3
  Logical Operator21/1 -> Logical Operator8/3
  Logical Operator22/1 -> Logical Operator7/2
  Logical Operator23/1 -> Logical Operator4/1
  Logical Operator24/1 -> Logical Operator2/1
  In_a/1 -> Logical Operator26/1, Logical Operator23/1, Logical Operator7/1, Logical Operator8/1, Logical Operator16/1, Logical Operator14/1, Logical Operator24/1, Logical Operator11/1
  Logical Operator25/1 -> Logical Operator2/3
  Logical Operator26/1 -> Logical Operator3/1
  Logical Operator27/1 -> Logical Operator3/2
  In_b/1 -> Logical Operator12/1, Logical Operator2/2, Logical Operator27/1, Logical Operator4/2, Logical Operator22/1, Logical Operator8/2, Logical Operator16/2, Logical Operator14/2
  only_K1/1 -> Logical Operator19/1, Logical Operator9/1
  only_K2/1 -> Logical Operator18/1, Logical Operator10/1
  only_K3/1 -> Logical Operator15/1, Logical Operator20/1
  Logical Operator17/1 -> 1/2
  1/1 -> out/1
  Logical Operator13/1 -> 1/3
  Logical Operator16/1 -> 1/1
  In_ c/1 -> Logical Operator1/1, Logical Operator25/1, Logical Operator3/3, Logical Operator4/3, Logical Operator7/3, Logical Operator21/1, Logical Operator16/3, Logical Operator14/3

== system mylib/264_DZ_trans_st_v1/St3/Subsystem ==
  T_fast_time : Inport
  T_fast_zero : Inport  Port=2
  "In1 " : Inport  Port=3
  "In2 " : Inport  Port=4
  "In3 " : Inport  Port=5
  {1..5,7} (6 alike) : Switch  Criteria=u2 > Threshold
  T1 : powerlib_meascontrol/Logic/On Delay  DelayType=On delay  delay=T_st  ic=0  Ts=0
  T2 : powerlib_meascontrol/Logic/On Delay  DelayType=On delay  delay=T_st  ic=0  Ts=0
  T3 : powerlib_meascontrol/Logic/On Delay  DelayType=On delay  delay=T_st  ic=0  Ts=0
  T4 : powerlib_meascontrol/Logic/On Delay  DelayType=On delay  delay=T_fast  ic=0  Ts=0
  T5 : powerlib_meascontrol/Logic/On Delay  DelayType=On delay  delay=T_fast  ic=0  Ts=0
  T6 : powerlib_meascontrol/Logic/On Delay  DelayType=On delay  delay=T_fast  ic=0  Ts=0
  T7 : powerlib_meascontrol/Logic/On Delay  DelayType=Off delay  delay=T_fast  ic=0  Ts=0
  Out1 : Outport
  Out2 : Outport  Port=2
  Out3 : Outport  Port=3
  wires:
  "In3 "/1 -> T4/1, T2/1, 4/1
  "In2 "/1 -> 3/1, T5/1, T1/1
  "In1 "/1 -> 5/1, T3/1, T6/1
  T7/1 -> 2/2, 1/2, 7/2
  T_fast_time/1 -> T7/1
  T4/1 -> 2/1
  T5/1 -> 1/1
  T6/1 -> 7/1
  T3/1 -> 7/3
  T1/1 -> 1/3
  T2/1 -> 2/3
  T_fast_zero/1 -> 5/2, 3/2, 4/2
  7/1 -> 5/3
  1/1 -> 3/3
  2/1 -> 4/3
  5/1 -> Out1/1
  3/1 -> Out2/1
  4/1 -> Out3/1

== system mylib/264_DZ_trans_st_v1/St3/in_1 ==
  jmp_in_zone : Inport
  in : Inport  Port=2
  jmp : Inport  Port=3
  1 : Switch  Criteria=u2 > Threshold
  10 : Logic  AllPortsSameDT=off  OutDataTypeStr=boolean
  11 : Logic  Operator=NOT  AllPortsSameDT=off  OutDataTypeStr=boolean
  12 : Memory
  3 : Logic  AllPortsSameDT=off  OutDataTypeStr=boolean
  RS : $bdroot/RS  SystemSampleTime=-1  Latency=0  AutoFrameSizeCalculation=off
  R_TRIG : $bdroot/R_TRIG  SystemSampleTime=-1  Latency=0  AutoFrameSizeCalculation=off
  T1 : powerlib_meascontrol/Logic/On Delay  DelayType=Off delay  delay=T_reset  ic=0  Ts=0
  T2 : powerlib_meascontrol/Logic/On Delay  DelayType=On delay  delay=T_reset  ic=0  Ts=0
  Y : Outport
  wires:
  RS/1 -> 12/1, Y/1
  in/1 -> 11/1, R_TRIG/1, 1/3
  R_TRIG/1 -> 1/1
  jmp_in_zone/1 -> 1/2
  11/1 -> 10/2
  10/1 -> T2/1
  T1/1 -> 3/2
  1/1 -> 3/1
  jmp/1 -> T1/1
  12/1 -> 10/1
  T2/1 -> RS/2
  3/1 -> RS/1

== system mylib/264_DZ_trans_st_v1/St3/in_2 ==
  jmp_in_zone : Inport
  in : Inport  Port=2
  jmp : Inport  Port=3
  1 : Switch  Criteria=u2 > Threshold
  10 : Logic  AllPortsSameDT=off  OutDataTypeStr=boolean
  11 : Logic  Operator=NOT  AllPortsSameDT=off  OutDataTypeStr=boolean
  12 : Memory
  3 : Logic  AllPortsSameDT=off  OutDataTypeStr=boolean
  RS : $bdroot/RS  SystemSampleTime=-1  Latency=0  AutoFrameSizeCalculation=off
  R_TRIG : $bdroot/R_TRIG  SystemSampleTime=-1  Latency=0  AutoFrameSizeCalculation=off
  T1 : powerlib_meascontrol/Logic/On Delay  DelayType=Off delay  delay=T_reset  ic=0  Ts=0
  T2 : powerlib_meascontrol/Logic/On Delay  DelayType=On delay  delay=T_reset  ic=0  Ts=0
  Y : Outport
  wires:
  RS/1 -> 12/1, Y/1
  in/1 -> 11/1, R_TRIG/1, 1/3
  R_TRIG/1 -> 1/1
  jmp_in_zone/1 -> 1/2
  11/1 -> 10/2
  10/1 -> T2/1
  T1/1 -> 3/2
  1/1 -> 3/1
  jmp/1 -> T1/1
  12/1 -> 10/1
  T2/1 -> RS/2
  3/1 -> RS/1

== system mylib/264_DZ_trans_st_v1/St3/in_3 ==
  jmp_in_zone : Inport
  in : Inport  Port=2
  jmp : Inport  Port=3
  1 : Switch  Criteria=u2 > Threshold
  10 : Logic  AllPortsSameDT=off  OutDataTypeStr=boolean
  11 : Logic  Operator=NOT  AllPortsSameDT=off  OutDataTypeStr=boolean
  12 : Memory
  3 : Logic  AllPortsSameDT=off  OutDataTypeStr=boolean
  RS : $bdroot/RS  SystemSampleTime=-1  Latency=0  AutoFrameSizeCalculation=off
  R_TRIG : $bdroot/R_TRIG  SystemSampleTime=-1  Latency=0  AutoFrameSizeCalculation=off
  T1 : powerlib_meascontrol/Logic/On Delay  DelayType=Off delay  delay=T_reset  ic=0  Ts=0
  T2 : powerlib_meascontrol/Logic/On Delay  DelayType=On delay  delay=T_reset  ic=0  Ts=0
  Y : Outport
  wires:
  RS/1 -> 12/1, Y/1
  in/1 -> 11/1, R_TRIG/1, 1/3
  R_TRIG/1 -> 1/1
  jmp_in_zone/1 -> 1/2
  11/1 -> 10/2
  10/1 -> T2/1
  T1/1 -> 3/2
  1/1 -> 3/1
  jmp/1 -> T1/1
  12/1 -> 10/1
  T2/1 -> RS/2
  3/1 -> RS/1

== system mylib/264_DZ_trans_st_v1/St3/k_type ==
  In_a : Inport
  In_b : Inport  Port=2
  In_ c : Inport  Port=3
  only_K1 : Inport  Port=4
  only_K2 : Inport  Port=5
  only_K3 : Inport  Port=6
  1 : Switch  Criteria=u2 > Threshold
  Logical Operator{1,12,18..27} (12 alike) : Logic  Operator=NOT  AllPortsSameDT=off  OutDataTypeStr=boolean
  Logical Operator10 : Logic  AllPortsSameDT=off  OutDataTypeStr=boolean
  Logical Operator{2..4,7..8,11,14,17} (8 alike) : Logic  Inputs=3  AllPortsSameDT=off  OutDataTypeStr=boolean
  Logical Operator{5..6,13,16} (4 alike) : Logic  Operator=OR  Inputs=3  AllPortsSameDT=off  OutDataTypeStr=boolean
  Logical Operator15 : Logic  AllPortsSameDT=off  OutDataTypeStr=boolean
  Logical Operator9 : Logic  AllPortsSameDT=off  OutDataTypeStr=boolean
  out : Outport
  wires:
  Logical Operator12/1 -> Logical Operator11/2
  Logical Operator1/1 -> Logical Operator11/3
  Logical Operator2/1 -> Logical Operator5/2
  Logical Operator11/1 -> Logical Operator5/1
  Logical Operator3/1 -> Logical Operator5/3
  Logical Operator4/1 -> Logical Operator6/1
  Logical Operator7/1 -> Logical Operator6/2
  Logical Operator8/1 -> Logical Operator6/3
  Logical Operator5/1 -> Logical Operator9/2
  Logical Operator6/1 -> Logical Operator10/2
  Logical Operator9/1 -> Logical Operator13/1
  Logical Operator10/1 -> Logical Operator13/2
  Logical Operator15/1 -> Logical Operator13/3
  Logical Operator14/1 -> Logical Operator15/2
  Logical Operator19/1 -> Logical Operator17/1
  Logical Operator18/1 -> Logical Operator17/2
  Logical Operator20/1 -> Logical Operator17/3
  Logical Operator21/1 -> Logical Operator8/3
  Logical Operator22/1 -> Logical Operator7/2
  Logical Operator23/1 -> Logical Operator4/1
  Logical Operator24/1 -> Logical Operator2/1
  In_a/1 -> Logical Operator26/1, Logical Operator23/1, Logical Operator7/1, Logical Operator8/1, Logical Operator16/1, Logical Operator14/1, Logical Operator24/1, Logical Operator11/1
  Logical Operator25/1 -> Logical Operator2/3
  Logical Operator26/1 -> Logical Operator3/1
  Logical Operator27/1 -> Logical Operator3/2
  In_b/1 -> Logical Operator12/1, Logical Operator2/2, Logical Operator27/1, Logical Operator4/2, Logical Operator22/1, Logical Operator8/2, Logical Operator16/2, Logical Operator14/2
  only_K1/1 -> Logical Operator19/1, Logical Operator9/1
  only_K2/1 -> Logical Operator18/1, Logical Operator10/1
  only_K3/1 -> Logical Operator15/1, Logical Operator20/1
  Logical Operator17/1 -> 1/2
  1/1 -> out/1
  Logical Operator13/1 -> 1/3
  Logical Operator16/1 -> 1/1
  In_ c/1 -> Logical Operator1/1, Logical Operator25/1, Logical Operator3/3, Logical Operator4/3, Logical Operator7/3, Logical Operator21/1, Logical Operator16/3, Logical Operator14/3

== system mylib/264_DZ_trans_st_v1/z_calc_ph_line19/R_lin_recalc ==
  R_a : Inport
  X_a : Inport  Port=2
  R_b : Inport  Port=3
  X_b : Inport  Port=4
  R_c : Inport  Port=5
  X_c : Inport  Port=6
  recalc_a : Inport  Port=7
  recalc_b : Inport  Port=8
  recalc_c : Inport  Port=9
  R_to_X : Inport  Port=10
  Divide10 : Product  Inputs=**
  Divide8 : Product  Inputs=**
  Divide9 : Product  Inputs=**
  Switch : Switch  Criteria=u2 > Threshold
  Switch1 : Switch  Criteria=u2 > Threshold
  Switch2 : Switch  Criteria=u2 > Threshold
  Ra : Outport
  Xa : Outport  Port=2
  Rb : Outport  Port=3
  Xb : Outport  Port=4
  Rc : Outport  Port=5
  Xc : Outport  Port=6
  wires:
  Divide8/1 -> Switch/1
  Divide9/1 -> Switch1/1
  Divide10/1 -> Switch2/1
  R_to_X/1 -> Divide10/2, Divide9/2, Divide8/2
  recalc_a/1 -> Switch2/2
  recalc_b/1 -> Switch1/2
  recalc_c/1 -> Switch/2
  X_c/1 -> Xc/1, Divide8/1
  X_b/1 -> Xb/1, Divide9/1
  X_a/1 -> Divide10/1, Xa/1
  R_a/1 -> Switch2/3
  R_b/1 -> Switch1/3
  R_c/1 -> Switch/3
  Switch1/1 -> Rb/1
  Switch2/1 -> Ra/1
  Switch/1 -> Rc/1

== system mylib/264_DZ_trans_st_v1/z_calc_ph_line19/R_ph_recalc ==
  R_a : Inport
  X_a : Inport  Port=2
  R_b : Inport  Port=3
  X_b : Inport  Port=4
  R_c : Inport  Port=5
  X_c : Inport  Port=6
  recalc_a : Inport  Port=7
  recalc_b : Inport  Port=8
  recalc_c : Inport  Port=9
  R_to_X : Inport  Port=10
  Divide10 : Product  Inputs=**
  Divide8 : Product  Inputs=**
  Divide9 : Product  Inputs=**
  Switch : Switch  Criteria=u2 > Threshold
  Switch1 : Switch  Criteria=u2 > Threshold
  Switch2 : Switch  Criteria=u2 > Threshold
  Ra : Outport
  Xa : Outport  Port=2
  Rb : Outport  Port=3
  Xb : Outport  Port=4
  Rc : Outport  Port=5
  Xc : Outport  Port=6
  wires:
  Divide8/1 -> Switch/1
  Divide9/1 -> Switch1/1
  Divide10/1 -> Switch2/1
  R_to_X/1 -> Divide10/2, Divide9/2, Divide8/2
  recalc_a/1 -> Switch2/2
  recalc_b/1 -> Switch1/2
  recalc_c/1 -> Switch/2
  X_c/1 -> Xc/1, Divide8/1
  X_b/1 -> Xb/1, Divide9/1
  X_a/1 -> Divide10/1, Xa/1
  R_a/1 -> Switch2/3
  R_b/1 -> Switch1/3
  R_c/1 -> Switch/3
  Switch1/1 -> Rb/1
  Switch2/1 -> Ra/1
  Switch/1 -> Rc/1

== system mylib/264_DZ_trans_st_v1/z_calc_ph_line19/Z_comp ==
  Ua_re : Inport
  Ua_im : Inport  Port=2
  Ub_re : Inport  Port=3
  Ub_im : Inport  Port=4
  Uc_re : Inport  Port=5
  Uc_im : Inport  Port=6
  Ia_re : Inport  Port=7
  Ia_im : Inport  Port=8
  Ib_re : Inport  Port=9
  Ib_im : Inport  Port=10
  Ic_re : Inport  Port=11
  Ic_im : Inport  Port=12
  I0_re_prl : Inport  Port=13
  I0_im_prl : Inport  Port=14
  K_I0_re : Inport  Port=15
  K_I0_im : Inport  Port=16
  K_I0_prl_re : Inport  Port=17
  K_I0_prl_im : Inport  Port=18
  Add : Sum  Inputs=+-
  Add1 : Sum  Inputs=+-
  Add2 : Sum  Inputs=+-
  Logical Operator{,1..5} (6 alike) : Logic  AllPortsSameDT=off  OutDataTypeStr=boolean
  Logical Operator6 : Logic  Operator=OR  AllPortsSameDT=off  OutDataTypeStr=boolean
  Logical Operator7 : Logic  Operator=OR  AllPortsSameDT=off  OutDataTypeStr=boolean
  Logical Operator8 : Logic  Operator=OR  AllPortsSameDT=off  OutDataTypeStr=boolean
  Max : MinMax  Function=max  Inputs=3
  Max1 : MinMax  Inputs=3
  Max2 : MinMax  Inputs=3
  Relational Operator{,1..8} (9 alike) : RelationalOperator  Operator===  OutDataTypeStr=boolean  RndMeth=Simplest
  Switch{,1..5} (6 alike) : Switch  Criteria=u2 > Threshold
  Z_a : Subsystem
  Z_b : Subsystem
  Z_c : Subsystem
  simpcomp : $bdroot/simpcomp  SystemSampleTime=-1  Latency=0  AutoFrameSizeCalculation=off
  Ra : Outport
  Xa : Outport  Port=2
  Rb : Outport  Port=3
  Xb : Outport  Port=4
  Rc : Outport  Port=5
  Xc : Outport  Port=6
  wires:
  Ia_re/1 -> Z_a/3(I_re), simpcomp/1
  Ia_im/1 -> Z_a/4(I_im), simpcomp/2
  Ib_re/1 -> Z_b/3(I_re), simpcomp/3
  Ib_im/1 -> Z_b/4(I_im), simpcomp/4
  Ic_re/1 -> Z_c/3(I_re), simpcomp/5
  Ic_im/1 -> Z_c/4(I_im), simpcomp/6
  Add1/1 -> Relational Operator1/2, Max2/2
  Add/1 -> Relational Operator/2, Max2/1
  Add2/1 -> Relational Operator2/2, Max2/3
  Max2/1 -> Relational Operator2/1, Relational Operator1/1, Relational Operator/1
  Max/1 -> Relational Operator5/1, Relational Operator4/1, Relational Operator3/1
  Max1/1 -> Relational Operator8/1, Relational Operator7/1, Relational Operator6/1
  Logical Operator/1 -> Logical Operator6/1
  Logical Operator1/1 -> Logical Operator7/1
  Logical Operator2/1 -> Logical Operator8/1
  Logical Operator3/1 -> Logical Operator6/2
  Logical Operator4/1 -> Logical Operator7/2
  Logical Operator5/1 -> Logical Operator8/2
  Relational Operator6/1 -> Logical Operator3/1
  Relational Operator7/1 -> Logical Operator4/1
  Relational Operator8/1 -> Logical Operator5/1
  Relational Operator3/1 -> Logical Operator/1
  Relational Operator4/1 -> Logical Operator1/1
  Relational Operator5/1 -> Logical Operator2/1
  Relational Operator/1 -> Logical Operator5/2, Logical Operator2/2
  Relational Operator1/1 -> Logical Operator/2, Logical Operator3/2
  Relational Operator2/1 -> Logical Operator1/2, Logical Operator4/2
  Switch/1 -> Xc/1
  Switch1/1 -> Rc/1
  Switch2/1 -> Xb/1
  Switch3/1 -> Rb/1
  Switch4/1 -> Xa/1
  Switch5/1 -> Ra/1
  Logical Operator8/1 -> Switch1/2, Switch/2
  Logical Operator7/1 -> Switch2/2, Switch3/2
  Logical Operator6/1 -> Switch4/2, Switch5/2
  Ua_re/1 -> Z_a/1(U_re)
  Ua_im/1 -> Z_a/2(U_im)
  Ub_re/1 -> Z_b/1(U_re)
  Ub_im/1 -> Z_b/2(U_im)
  Uc_re/1 -> Z_c/1(U_re)
  Uc_im/1 -> Z_c/2(U_im)
  simpcomp/2 -> Z_c/6(I0_im), Z_b/6(I0_im), Z_a/6(I0_im)
  simpcomp/1 -> Z_c/5(I0_re), Z_b/5(I0_re), Z_a/5(I0_re)
  I0_re_prl/1 -> Z_c/7(I0_re_prl), Z_b/7(I0_re_prl), Z_a/7(I0_re_prl)
  I0_im_prl/1 -> Z_c/8(I0_im_prl), Z_b/8(I0_im_prl), Z_a/8(I0_im_prl)
  K_I0_re/1 -> Z_b/9(K_I0_re), Z_a/9(K_I0_re), Z_c/9(K_I0_re)
  K_I0_im/1 -> Z_c/10(K_I0_im), Z_b/10(K_I0_im), Z_a/10(K_I0_im)
  K_I0_prl_re/1 -> Z_c/11(K_I0_prl_re), Z_b/11(K_I0_prl_re), Z_a/11(K_I0_prl_re)
  K_I0_prl_im/1 -> Z_b/12(K_I0_prl_im), Z_a/12(K_I0_prl_im), Z_c/12(K_I0_prl_im)
  Z_c/6(Z) -> Max/3, Relational Operator5/2, Add2/2, Add1/2, Max1/3, Relational Operator8/2
  Z_b/6(Z) -> Max/2, Add1/1, Add/2, Relational Operator4/2, Relational Operator7/2, Max1/2
  Z_a/6(Z) -> Add2/1, Add/1, Relational Operator3/2, Max/1, Relational Operator6/2, Max1/1
  Z_c/3(X_comp) -> Switch/3
  Z_c/4(X) -> Switch/1
  Z_b/3(X_comp) -> Switch2/3
  Z_b/4(X) -> Switch2/1
  Z_b/1(R_comp) -> Switch3/3
  Z_c/1(R_comp) -> Switch1/3
  Z_c/2(R) -> Switch1/1
  Z_b/2(R) -> Switch3/1
  Z_a/1(R_comp) -> Switch5/3
  Z_a/3(X_comp) -> Switch4/3
  Z_a/2(R) -> Switch5/1
  Z_a/4(X) -> Switch4/1

== system mylib/264_DZ_trans_st_v1/z_calc_ph_line19/Z_lin ==
  Ua_re : Inport
  Ua_im : Inport  Port=2
  Ub_re : Inport  Port=3
  Ub_im : Inport  Port=4
  Uc_re : Inport  Port=5
  Uc_im : Inport  Port=6
  Ia_re : Inport  Port=7
  Ia_im : Inport  Port=8
  Ib_re : Inport  Port=9
  Ib_im : Inport  Port=10
  Ic_re : Inport  Port=11
  Ic_im : Inport  Port=12
  det_K2_ab : Inport  Port=13
  det_K2_bc : Inport  Port=14
  det_K2_ca : Inport  Port=15
  Z_ab : Subsystem
  Z_bc : Subsystem
  Z_ca : Subsystem
  Rab : Outport
  Xab : Outport  Port=2
  Rbc : Outport  Port=3
  Xbc : Outport  Port=4
  Rca : Outport  Port=5
  Xca : Outport  Port=6
  wires:
  Z_ab/1(R) -> Rab/1
  Z_ab/2(X) -> Xab/1
  Z_ca/1(R) -> Rca/1
  Z_ca/2(X) -> Xca/1
  Z_bc/2(X) -> Xbc/1
  Z_bc/1(R) -> Rbc/1
  Ua_re/1 -> Z_ab/1(U_ph1_re), Z_ca/3(U_ph2_re)
  Ua_im/1 -> Z_ab/2(U_ph1_im), Z_ca/4(U_ph2_im)
  Ub_re/1 -> Z_ab/3(U_ph2_re), Z_bc/1(U_ph1_re)
  Ub_im/1 -> Z_ab/4(U_ph2_im), Z_bc/2(U_ph1_im)
  Uc_re/1 -> Z_ca/1(U_ph1_re), Z_bc/3(U_ph2_re)
  Uc_im/1 -> Z_ca/2(U_ph1_im), Z_bc/4(U_ph2_im)
  Ia_re/1 -> Z_ab/5(I_ph1_re), Z_ca/7(I_ph2_re)
  Ia_im/1 -> Z_ab/6(I_ph1_im), Z_ca/8(I_ph2_im)
  Ib_re/1 -> Z_bc/5(I_ph1_re), Z_ab/7(I_ph2_re)
  Ib_im/1 -> Z_ab/8(I_ph2_im), Z_bc/6(I_ph1_im)
  Ic_re/1 -> Z_ca/5(I_ph1_re), Z_bc/7(I_ph2_re)
  Ic_im/1 -> Z_ca/6(I_ph1_im), Z_bc/8(I_ph2_im)
  det_K2_ab/1 -> Z_ab/9(det_K2)
  det_K2_bc/1 -> Z_bc/9(det_K2)
  det_K2_ca/1 -> Z_ca/9(det_K2)

== system mylib/264_DZ_trans_st_v1/z_calc_ph_line19/det_k2 ==
  Ua_re1 : Inport
  Ua_im1 : Inport  Port=2
  Ub_re1 : Inport  Port=3
  Ub_im1 : Inport  Port=4
  Uc_re1 : Inport  Port=5
  Uc_im1 : Inport  Port=6
  in_range_Ua : Inport  Port=7
  in_range_Ub : Inport  Port=8
  in_range_Uc : Inport  Port=9
  in_range_Uab : Inport  Port=10
  in_range_Ubc : Inport  Port=11
  in_range_Uca : Inport  Port=12
  arg_U_K2 : Inport  Port=13
  Logical Operator{6..11,15..17} (9 alike) : Logic  AllPortsSameDT=off  OutDataTypeStr=boolean
  Logical Operator12 : Logic  Operator=NOT  AllPortsSameDT=off  OutDataTypeStr=boolean
  Logical Operator13 : Logic  Operator=NOT  AllPortsSameDT=off  OutDataTypeStr=boolean
  Logical Operator14 : Logic  Operator=NOT  AllPortsSameDT=off  OutDataTypeStr=boolean
  Relational Operator6 : RelationalOperator  Operator=<  OutDataTypeStr=boolean  RndMeth=Simplest
  Relational Operator7 : RelationalOperator  Operator=<  OutDataTypeStr=boolean  RndMeth=Simplest
  Relational Operator8 : RelationalOperator  Operator=<  OutDataTypeStr=boolean  RndMeth=Simplest
  ab_arg : $bdroot/delta_calc  SystemSampleTime=-1  Latency=0  AutoFrameSizeCalculation=off
  bc_arg : $bdroot/delta_calc  SystemSampleTime=-1  Latency=0  AutoFrameSizeCalculation=off
  ca_arg : $bdroot/delta_calc  SystemSampleTime=-1  Latency=0  AutoFrameSizeCalculation=off
  det_K2_ab : Outport
  det_K2_bc : Outport  Port=2
  det_K2_ca : Outport  Port=3
  wires:
  Relational Operator8/1 -> Logical Operator17/1
  Ub_im1/1 -> ab_arg/4, bc_arg/2
  in_range_Ua/1 -> Logical Operator8/2, Logical Operator6/1
  Ua_im1/1 -> ab_arg/2, ca_arg/4
  Uc_re1/1 -> bc_arg/3, ca_arg/1
  arg_U_K2/1 -> Relational Operator6/2, Relational Operator7/2, Relational Operator8/2
  Uc_im1/1 -> bc_arg/4, ca_arg/2
  ab_arg/1 -> Relational Operator6/1  "Ia_re"
  in_range_Ub/1 -> Logical Operator7/1, Logical Operator6/2
  Ub_re1/1 -> ab_arg/3, bc_arg/1
  Logical Operator14/1 -> Logical Operator9/2
  Logical Operator17/1 -> Logical Operator11/1
  in_range_Uab/1 -> Logical Operator14/1
  Logical Operator15/1 -> Logical Operator9/1
  Relational Operator7/1 -> Logical Operator16/1
  Logical Operator8/1 -> Logical Operator17/2
  in_range_Uc/1 -> Logical Operator7/2, Logical Operator8/1
  in_range_Ubc/1 -> Logical Operator13/1
  Ua_re1/1 -> ab_arg/1, ca_arg/3
  Logical Operator12/1 -> Logical Operator11/2
  Logical Operator10/1 -> det_K2_bc/1
  Logical Operator13/1 -> Logical Operator10/2
  Relational Operator6/1 -> Logical Operator15/1
  Logical Operator16/1 -> Logical Operator10/1
  Logical Operator6/1 -> Logical Operator15/2
  in_range_Uca/1 -> Logical Operator12/1
  Logical Operator7/1 -> Logical Operator16/2
  bc_arg/1 -> Relational Operator7/1  "Ia_re"
  Logical Operator11/1 -> det_K2_ca/1
  ca_arg/1 -> Relational Operator8/1  "Ia_re"
  Logical Operator9/1 -> det_K2_ab/1
